simulink model "model4_3"
settings: Solver=ode4  SolverMode=SingleTasking  StartTime=0.0  StopTime=1000.0  FixedStep=0.01  RelTol=1e-3
values from neighbouring files (symbols this model uses):
  a1 = 2    [lab4_3_2.m]
  a2 = 3    [lab4_3_2.m]
  a3 = 1    [lab4_3_2.m]
  a4 = 2    [lab4_3_2.m]
  a5 = 4    [lab4_3_2.m]
  p1 = 1    [lab4_3_2.m]
  p2 = 5    [lab4_3_2.m]
  p3 = 2    [lab4_3_2.m]
  p4 = 1    [lab4_3_2.m]
  p5 = 0    [lab4_3_2.m]
  w1 = 0.001    [lab4_3_2.m]
  w2 = 1    [lab4_3_2.m]
  w3 = 30    [lab4_3_2.m]
  w4 = 0.01    [lab4_3_2.m]
  w5 = 5    [lab4_3_2.m]
settings Model: Creator=Dell  LastModifiedBy=student
settings DataIOCC: LimitDataPoints=on  SaveFormat=Array  SignalLoggingSaveFormat=ModelDataLogs  ReturnWorkspaceOutputs=off
settings OptimizationCC: BlockReduction=off  BooleanDataType=off  ExpressionDepthLimit=2147483647  LifeSpan=inf  SimCompilerOptimization=Off
settings DebuggingCC: SaveWithParameterizedLinksMsg=none  UnderspecifiedInitializationDetection=Classic  MergeDetectMultiDrivingBlocksExec=none  SignalResolutionControl=TryResolveAllWithWarning  MultiTaskDSMMsg=warning  MultiTaskCondExecSysMsg=none  FcnCallInpInsideContextMsg=Enable All  FrameProcessingCompatibilityMsg=warning  StateNameClashWarn=warning  StrictBusMsg=None  SFUnexpectedBacktrackingDiag=warning  SFNoUnconditionalDefaultTransitionDiag=warning
settings HardwareCC: ProdBitPerPointer=32  ProdLargestAtomicFloat=None  ProdIntDivRoundTo=Undefined  ProdEndianess=Unspecified  ProdWordSize=32  ProdHWDeviceType=32-bit Generic  TargetUnknown=on
settings ModelReferenceCC: PropagateSignalLabelsOutOfModel=off
settings SFSimCC: SimUseLocalCustomCode=off
settings RTWCC: RTWUseLocalCustomCode=off  IncludeERTFirstTime=on  RTWCompilerOptimization=Off
settings CodeAppCC: CustomSymbolStrType=$N$R$M
settings GRTTargetCC: CodeReplacementLibrary=ANSI_C  GeneratePreprocessorConditionals=Disable all  CPPClassGenCompliant=off

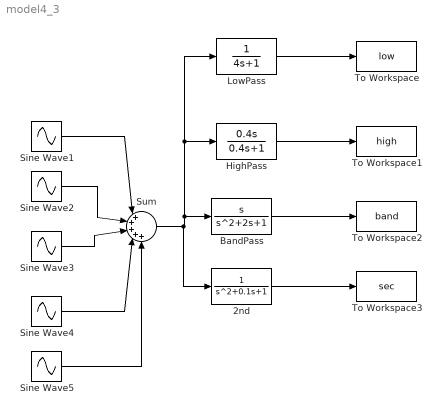
== system model4_3 ==
  2nd : TransferFcn  Denominator=[1 0.1 1]
  BandPass : TransferFcn  Numerator=[1 0]
  HighPass : TransferFcn  Numerator=[0.4 0]  Denominator=[0.4 1]
  LowPass : TransferFcn  Denominator=[4 1]
  Sine Wave1 : Sin  Amplitude=a1  Frequency=w1  Phase=p1  SampleTime=0
  Sine Wave2 : Sin  Amplitude=a2  Frequency=w2  Phase=p2  SampleTime=0
  Sine Wave3 : Sin  Amplitude=a3  Frequency=w3  Phase=p3  SampleTime=0
  Sine Wave4 : Sin  Amplitude=a4  Frequency=w4  Phase=p4  SampleTime=0
  Sine Wave5 : Sin  Amplitude=a5  Frequency=w5  Phase=p5  SampleTime=0
  Sum : Sum  Inputs=|+++++
  To Workspace : ToWorkspace  VariableName=low  SampleTime=-1  SaveFormat=Timeseries
  To Workspace1 : ToWorkspace  VariableName=high  SampleTime=-1  SaveFormat=Timeseries
  To Workspace2 : ToWorkspace  VariableName=band  SampleTime=-1  SaveFormat=Timeseries
  To Workspace3 : ToWorkspace  VariableName=sec  SampleTime=-1  SaveFormat=Timeseries
  wires:
  LowPass/1 -> To Workspace/1
  HighPass/1 -> To Workspace1/1
  BandPass/1 -> To Workspace2/1
  2nd/1 -> To Workspace3/1
  Sine Wave1/1 -> Sum/1
  Sine Wave2/1 -> Sum/2
  Sine Wave3/1 -> Sum/3
  Sine Wave4/1 -> Sum/4
  Sine Wave5/1 -> Sum/5
  Sum/1 -> 2nd/1, LowPass/1, HighPass/1, BandPass/1
